simulink model "dc_motor_model"  (R2023b)
settings: Solver=VariableStepAuto  StartTime=0.0  StopTime=10.0  RelTol=1e-3
undefined symbols (not defined in the file or in its folder): b, J, K, L, R
settings Model: Creator=berkeozener  LastModifiedBy=berkeozener

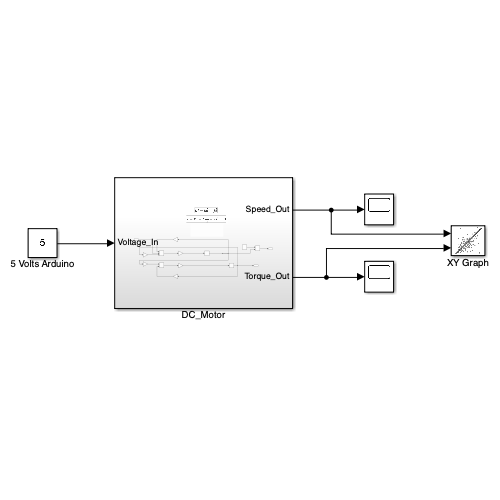
[thumbnail: Simulink's stored preview of the top-level diagram]
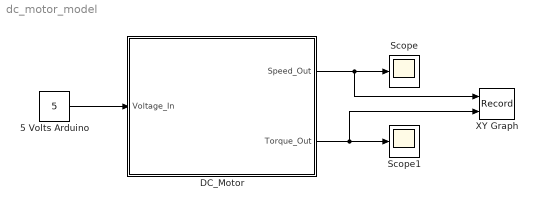
== system dc_motor_model ==
  5 Volts Arduino : Constant  Value=5
  DC_Motor : Subsystem
  Scope : Scope
  Scope1 : Scope
  XY Graph : Record  FileSettingsInternal="{\"entries\":[{\"content\":{\"excelSettings\":{\"content\":{},\"type\":\"Streamout.ExcelSettings\"}},\"type\":\"Streamout.FileSettingStorage\",\"uuid\":\"\"}],\"packageUris\":[\"http:\\/\\/schema.mathworks.com\\/mf0\\/streamout_blocks\\/R2020a\"],\"version\":\"1.0\"}"  Layout=[1 1]  SignalsInternal="{\"entries\":[{\"content\":{\"signals\":[{\"content\":{\"blockPath\":[],\"dimensions\":[1],\"domain\":\"\",\"lineColor\":\"#a2142f\",\"plots\":[ 1 ],\"port\":1,\"sid\":[\"\"],\"signalID\":1,\"signalName\":\"DC_Motor:1\"},\"type\":\"RecordBlkView.Signal\",\"uuid\":\"\"},{\"content\":{\"blockPath\":[],\"dimensions\":[1],\"domain\":\"\",\"lineColor\":\"#139fff\",\"plots\":[ 1 ],\"port\":2,\"sid\":[\"\"],\"signalID\":2,\"signalName\":\"DC_Motor:2\"},\"type\":\"RecordBlkView.Signal\",\"uuid\":\"\"}]},\"type\":\"RecordBlkView.InputSignals\",\"uuid\":\"\"}],\"packageUris\":[\"http:\\/\\/schema.mathworks.com\\/mf0\\/streamout_blocks\\/R2020a\"],\"version\":\"1.0\"}"  VisualizationBindings="{\"xyplotplugin\":{\"info\":[{\"series\":[{\"bindingParametersList\":[{\"parameter\":\"X-Axis\",\"signalID\":1,\"signalName\":\"DC_Motor:1\"},{\"parameter\":\"Y-Axis\",\"signalID\":2,\"signalName\":\"DC_Motor:2\"}],\"seriesID\":0}],\"subplotID\":1}]}}"  CompatibilityTag=XY
  wires:
  5 Volts Arduino/1 -> DC_Motor/1(Voltage_In)
  DC_Motor/1(Speed_Out) -> XY Graph/1, Scope/1
  DC_Motor/2(Torque_Out) -> XY Graph/2, Scope1/1

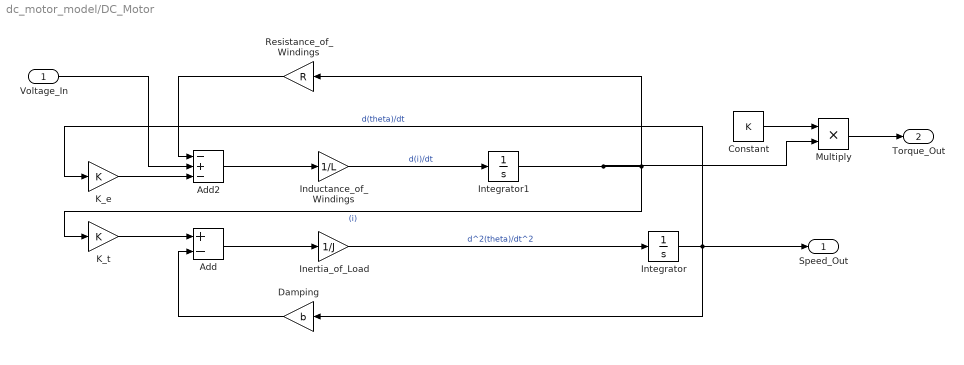
== system dc_motor_model/DC_Motor ==
  Voltage_In : Inport
  Add : Sum  Inputs=+-
  Add2 : Sum  Inputs=-+-
  Constant : Constant  Value=K
  Damping : Gain  Gain=b
  Inductance_of_Windings : Gain  Gain=1/L
  Inertia_of_Load : Gain  Gain=1/J
  Integrator : Integrator
  Integrator1 : Integrator
  K_e : Gain  Gain=K
  K_t : Gain  Gain=K
  Multiply : Product  Inputs=**
  Resistance_of_Windings : Gain  Gain=R
  Speed_Out : Outport
  Torque_Out : Outport  Port=2
  wires:
  Add/1 -> Inertia_of_Load/1
  Inertia_of_Load/1 -> Integrator/1  "d^2(theta)/dt^2"
  K_t/1 -> Add/1
  Add2/1 -> Inductance_of_Windings/1
  Resistance_of_Windings/1 -> Add2/1
  Integrator/1 -> Speed_Out/1, Damping/1, K_e/1  "d(theta)/dt"
  Voltage_In/1 -> Add2/2
  K_e/1 -> Add2/3
  Integrator1/1 -> Multiply/2, Resistance_of_Windings/1, K_t/1  "(i)"
  Inductance_of_Windings/1 -> Integrator1/1  "d(i)/dt"
  Damping/1 -> Add/2
  Multiply/1 -> Torque_Out/1
  Constant/1 -> Multiply/1
